simulink model "Mechanical"  (R2021a)
settings: Solver=VariableStepAuto  StartTime=0.0  StopTime=10.0  RelTol=1e-3
values from neighbouring files (symbols this model uses):
  Dm = 0.0071    [QuanserData.m]
  Dp = 0.0071    [QuanserData.m]
  Dt = 0.158    [QuanserData.m]
  g = 9.81    [QuanserData.m]
  Jeq = Jm+Jh+Jp    (= 1.120304e-05)    [QuanserData.m]
  Jp = 2.15e-2    (= 0.0215)    [QuanserData.m]
  k1 = 1.2e-5    (= 1.2e-05)    [QuanserData.m]
  k2 = 3.54e-9    (= 3.54e-09)    [QuanserData.m]
  k3 = -9.06e-5    (= -9.06e-05)    [QuanserData.m]
  k4 = 7.83e-7    (= 7.83e-07)    [QuanserData.m]
  km = 0.042    [QuanserData.m]
  Lm = 1.16e-3    (= 0.00116)    [QuanserData.m]
  Mb = 1.15    [QuanserData.m]
  Rm = 8.4    [QuanserData.m]
settings Model: Creator=y.briere  LastModifiedBy=fades
settings SolverCC: AlgebraicLoopSolver=TrustRegion
settings DataIOCC: InitialState=[]  LoadInitialState=on  ReturnWorkspaceOutputs=off
settings DebuggingCC: SFMachineParentedDataDiag=warning  ArithmeticOperatorsInVariantConditions=warning
settings SFSimCC: CustomCodeUndefinedFunction=UseInterfaceOnly

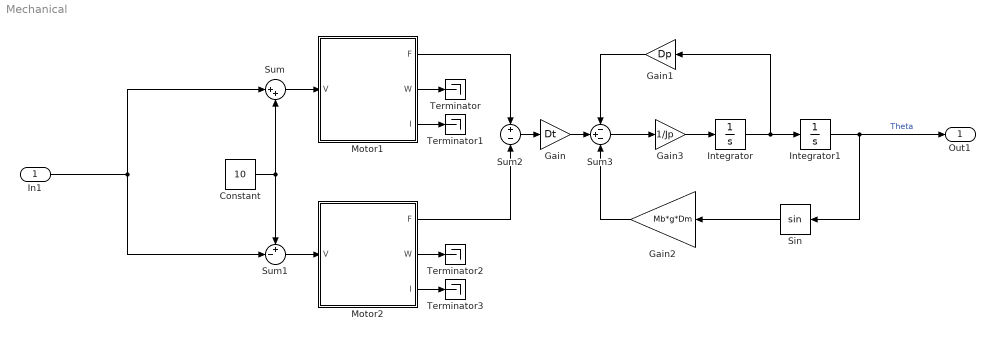
== system Mechanical ==
  In1 : Inport
  Constant : Constant  Value=10
  Gain : Gain  Gain=Dt
  Gain1 : Gain  Gain=Dp
  Gain2 : Gain  Gain=Mb*g*Dm
  Gain3 : Gain  Gain=1/Jp
  Integrator : Integrator
  Integrator1 : Integrator
  Motor1 : Subsystem
  Motor2 : Subsystem
  Sin : Trigonometry
  Sum : Sum  Inputs=|++
  Sum1 : Sum  Inputs=+-|
  Sum2 : Sum  Inputs=+-
  Sum3 : Sum  Inputs=-+-
  Terminator{,1..3} (4 alike) : Terminator
  Out1 : Outport  VectorParamsAs1DForOutWhenUnconnected=off
  wires:
  Sum1/1 -> Motor2/1(V)
  Sum/1 -> Motor1/1(V)
  Sum2/1 -> Gain/1
  Motor1/2(W) -> Terminator/1
  Motor1/3(I) -> Terminator1/1
  Motor2/2(W) -> Terminator2/1
  Motor2/3(I) -> Terminator3/1
  In1/1 -> Sum/1, Sum1/2
  Constant/1 -> Sum/2, Sum1/1
  Integrator1/1 -> Sin/1, Out1/1  "Theta"
  Gain/1 -> Sum3/2
  Gain1/1 -> Sum3/1
  Gain2/1 -> Sum3/3
  Sum3/1 -> Gain3/1
  Gain3/1 -> Integrator/1
  Integrator/1 -> Gain1/1, Integrator1/1
  Sin/1 -> Gain2/1
  Motor1/1(F) -> Sum2/1
  Motor2/1(F) -> Sum2/2

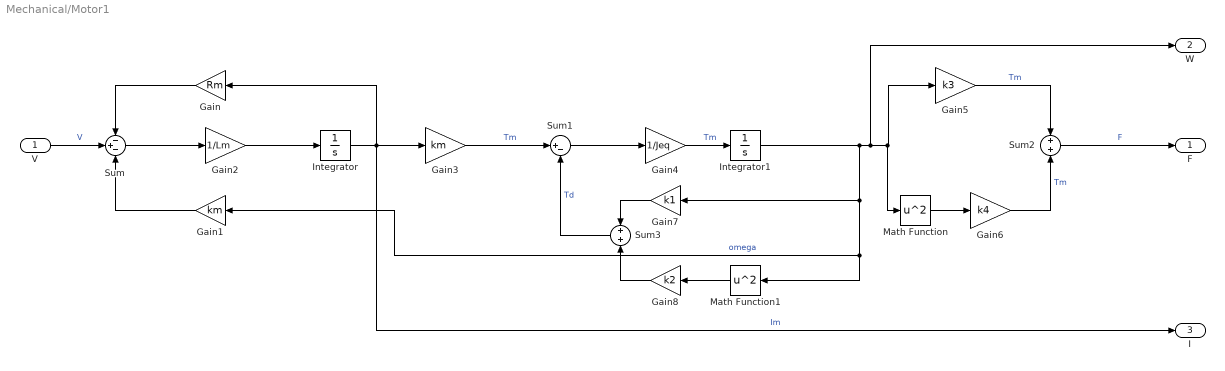
== system Mechanical/Motor1 ==
  V : Inport
  Gain : Gain  Gain=Rm
  Gain1 : Gain  Gain=km
  Gain2 : Gain  Gain=1/Lm
  Gain3 : Gain  Gain=km
  Gain4 : Gain  Gain=1/Jeq
  Gain5 : Gain  Gain=k3
  Gain6 : Gain  Gain=k4
  Gain7 : Gain  Gain=k1
  Gain8 : Gain  Gain=k2
  Integrator : Integrator
  Integrator1 : Integrator
  Math Function : Math  Operator=square  SaturateOnIntegerOverflow=on
  Math Function1 : Math  Operator=square  SaturateOnIntegerOverflow=on
  Sum : Sum  Inputs=-+-
  Sum1 : Sum  Inputs=|+-
  Sum2 : Sum
  Sum3 : Sum
  F : Outport  VectorParamsAs1DForOutWhenUnconnected=off
  W : Outport  Port=2  VectorParamsAs1DForOutWhenUnconnected=off
  I : Outport  Port=3  VectorParamsAs1DForOutWhenUnconnected=off
  wires:
  V/1 -> Sum/2  "V"
  Math Function1/1 -> Gain8/1
  Math Function/1 -> Gain6/1
  Gain7/1 -> Sum3/1
  Gain8/1 -> Sum3/2
  Gain5/1 -> Sum2/1  "Tm"
  Gain6/1 -> Sum2/2  "Tm"
  Integrator/1 -> I/1, Gain3/1, Gain/1  "Im"
  Sum2/1 -> F/1  "F"
  Gain2/1 -> Integrator/1
  Gain4/1 -> Integrator1/1  "Tm"
  Sum3/1 -> Sum1/2  "Td"
  Sum/1 -> Gain2/1
  Integrator1/1 -> Math Function1/1, Gain1/1, Gain7/1, W/1, Math Function/1, Gain5/1  "omega"
  Sum1/1 -> Gain4/1
  Gain3/1 -> Sum1/1  "Tm"
  Gain/1 -> Sum/1
  Gain1/1 -> Sum/3

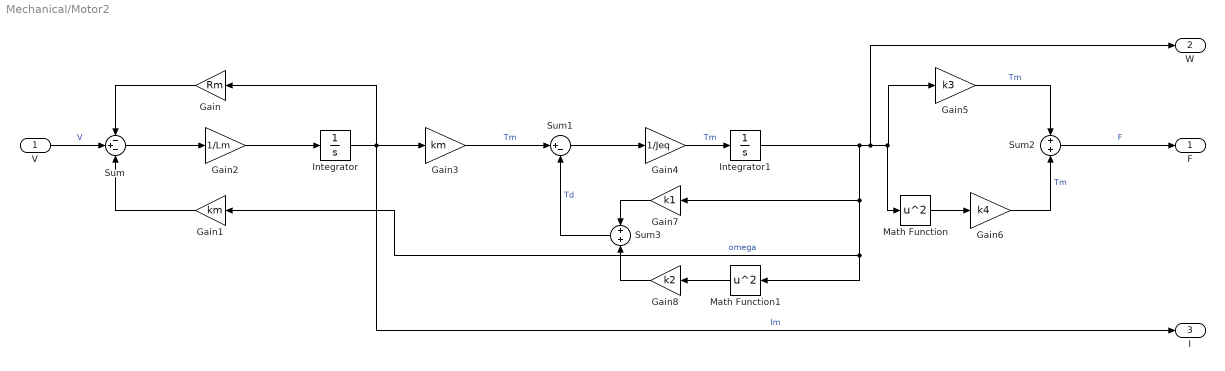
== system Mechanical/Motor2 ==
  V : Inport
  Gain : Gain  Gain=Rm
  Gain1 : Gain  Gain=km
  Gain2 : Gain  Gain=1/Lm
  Gain3 : Gain  Gain=km
  Gain4 : Gain  Gain=1/Jeq
  Gain5 : Gain  Gain=k3
  Gain6 : Gain  Gain=k4
  Gain7 : Gain  Gain=k1
  Gain8 : Gain  Gain=k2
  Integrator : Integrator
  Integrator1 : Integrator
  Math Function : Math  Operator=square  SaturateOnIntegerOverflow=on
  Math Function1 : Math  Operator=square  SaturateOnIntegerOverflow=on
  Sum : Sum  Inputs=-+-
  Sum1 : Sum  Inputs=|+-
  Sum2 : Sum
  Sum3 : Sum
  F : Outport  VectorParamsAs1DForOutWhenUnconnected=off
  W : Outport  Port=2  VectorParamsAs1DForOutWhenUnconnected=off
  I : Outport  Port=3  VectorParamsAs1DForOutWhenUnconnected=off
  wires:
  Gain7/1 -> Sum3/1
  Gain8/1 -> Sum3/2
  Gain5/1 -> Sum2/1  "Tm"
  Integrator/1 -> I/1, Gain3/1, Gain/1  "Im"
  Math Function1/1 -> Gain8/1
  V/1 -> Sum/2  "V"
  Math Function/1 -> Gain6/1
  Gain/1 -> Sum/1
  Gain1/1 -> Sum/3
  Gain3/1 -> Sum1/1  "Tm"
  Integrator1/1 -> Math Function1/1, Gain1/1, Gain7/1, W/1, Math Function/1, Gain5/1  "omega"
  Gain6/1 -> Sum2/2  "Tm"
  Sum3/1 -> Sum1/2  "Td"
  Sum/1 -> Gain2/1
  Gain2/1 -> Integrator/1
  Gain4/1 -> Integrator1/1  "Tm"
  Sum2/1 -> F/1  "F"
  Sum1/1 -> Gain4/1
